simulink library "FVT_lib"  (R2021b)
settings: Solver=VariableStepAuto  StartTime=0.0  StopTime=10.0  RelTol=1e-3
undefined symbols (not defined in the file): C_TASK_5MS_S, CANFDArray, ENUM_FAULTSTATE_FAIL, ENUM_FAULTSTATE_INDETERMINATE, ENUM_FAULTSTATE_PASS, EPSILON, FALSE, KHAL_CounterMAX_enum, KHAL_CounterMAXE2E_enum, LINArray, ONE_INT, TRUE, UNKNOWN, XX2KXX, ZERO_FLOAT, ZERO_INT
libraries: hdlsllib x41, simulink x23, hcu_lib x7, $bdroot x2
(part 2 of 3)

== system FVT_lib/hal/LIN_Scheduler ==
  Chart1 : Stateflow chart  TreatAsAtomicUnit=on
  Constant1 : Constant  Value=C_TASK_5MS_S
  Constant2 : Constant  Value=FirstDelayTime
  Constant3 : Constant  Value=C_TASK_5MS_S
  Constant4 : Constant  Value=CycleTime
  Data Type Conversion : DataTypeConversion  OutDataTypeStr=uint16
  Data Type Conversion1 : DataTypeConversion  OutDataTypeStr=uint16
  Divide : Product  Inputs=*/
  Divide1 : Product  Inputs=*/
  Gain : Gain  Gain=0.001
  Gain1 : Gain  Gain=0.001
  trig_LINReq : Outport
  wires:
  Data Type Conversion/1 -> Chart1/1(CycleCounter)
  Divide/1 -> Data Type Conversion1/1
  Chart1/1(trig_LINReq()) -> trig_LINReq/1
  Constant1/1 -> Divide/2
  Constant3/1 -> Divide1/2
  Divide1/1 -> Data Type Conversion/1
  Data Type Conversion1/1 -> Chart1/2(FirstDelayCounter)
  Constant4/1 -> Gain/1
  Gain/1 -> Divide1/1
  Constant2/1 -> Gain1/1
  Gain1/1 -> Divide/1

== system FVT_lib/hal/MessageRollingCounter ==
  Constant : Constant  Value=task_time_ms  OutDataTypeStr=uint16
  Constant1 : Constant  Value=msg_time_ms  OutDataTypeStr=uint16
  Constant2 : Constant  Value=ONE_INT
  Data Type Conversion : DataTypeConversion  OutDataTypeStr=uint16
  Data Type Conversion1 : DataTypeConversion  OutDataTypeStr=uint16
  Divide : Product  Inputs=*/  OutDataTypeStr=uint16
  Max : MinMax  Function=max  Inputs=2
  Scheduler : Stateflow chart  TreatAsAtomicUnit=on
  Subsystem : Subsystem
  out : Outport
  wires:
  Subsystem/1(RC) -> out/1
  Scheduler/1(trig_counter()) -> Subsystem/Trigger
  Constant1/1 -> Divide/1
  Constant/1 -> Max/1
  Max/1 -> Divide/2
  Constant2/1 -> Data Type Conversion/1
  Data Type Conversion/1 -> Max/2
  Divide/1 -> Data Type Conversion1/1
  Data Type Conversion1/1 -> Scheduler/1(counter_max)

== system FVT_lib/hal/MsgTimeoutJudge_CAN ==
  Rollcnt : Inport
  Constant : Constant  Value=C_TASK_5MS_S
  Constant1 : Constant  Value=1000  OutDataTypeStr=single
  Constant2 : Constant  Value=Gain
  Constant3 : Constant  Value=CycleTime
  Constant4 : Constant  Value=0.001
  DetectChange1 : Subsystem
      mask help: DetectChange
  Equal : RelationalOperator  Operator=>  OutDataTypeStr=boolean  RndMeth=Simplest
  NOT : Logic  Operator=NOT  AllPortsSameDT=off  OutDataTypeStr=boolean
  Product : Product
  Product1 : Product
  Timer1 : Subsystem  mask(Timer){}
      mask help: Timer funcion.
  MsgTimeout_flg : Outport
  wires:
  Rollcnt/1 -> DetectChange1/1(cnt)
  NOT/1 -> Timer1/1(trigger)
  DetectChange1/1(InValid) -> NOT/1, Timer1/2(reset)
  Constant1/1 -> Timer1/4(max_time)
  Constant/1 -> Timer1/3(Ts)
  Constant2/1 -> Product/2
  Product/1 -> Equal/2
  Timer1/1(time) -> Equal/1
  Equal/1 -> MsgTimeout_flg/1
  Constant3/1 -> Product1/1
  Constant4/1 -> Product1/2
  Product1/1 -> Product/1

== system FVT_lib/hal/MsgTimeoutJudge_CAN_AUTOSAR ==
  Cast To Boolean13 : DataTypeConversion  OutDataTypeStr=boolean
  Constant : Constant  Value=TRUE
  Latch13 : hcu_lib/Basic_Blocks/Latch
  Switch13 : Switch  Criteria=u2 ~= 0
  Unit Delay : UnitDelay  SampleTime=-1  HasFrameUpgradeWarning=on
  UnitConverter : DataTypeConversion  OutDataTypeStr=boolean
  Out : Outport
  wires:
  Latch13/1 -> Switch13/2
  Switch13/1 -> UnitConverter/1
  UnitConverter/1 -> Out/1, Unit Delay/1
  Cast To Boolean13/1 -> Latch13/1, Switch13/1
  Unit Delay/1 -> Cast To Boolean13/1
  Constant/1 -> Switch13/3

== system FVT_lib/hal/MsgTimeoutJudge_LIN ==
  Rollcnt : Inport
  Constant2 : Constant  Value=TimeoutCnt
  Data Type Conversion : DataTypeConversion  OutDataTypeStr=uint8
  Data Type Conversion1 : DataTypeConversion  OutDataTypeStr=uint8
  Equal : RelationalOperator  OutDataTypeStr=boolean  RndMeth=Simplest
  MsgTimeout_flg : Outport
  wires:
  Equal/1 -> MsgTimeout_flg/1
  Rollcnt/1 -> Data Type Conversion1/1
  Constant2/1 -> Data Type Conversion/1
  Data Type Conversion/1 -> Equal/2
  Data Type Conversion1/1 -> Equal/1

== system FVT_lib/hal/MsgTxController ==
  TxReq : Inport
  Chart : Stateflow chart  TreatAsAtomicUnit=on
  Constant : Constant  Value=C_TASK_5MS_S
  Constant3 : Constant  Value=CycleTime
  Data Type Conversion : DataTypeConversion  OutDataTypeStr=uint16
  Divide : Product  Inputs=*/
  Gain : Gain  Gain=0.001
  TxTrigger : Outport
  wires:
  Constant/1 -> Divide/2
  TxReq/1 -> Chart/1(TxReq)
  Divide/1 -> Data Type Conversion/1
  Chart/1(TxTrigger()) -> TxTrigger/1
  Gain/1 -> Divide/1
  Constant3/1 -> Gain/1
  Data Type Conversion/1 -> Chart/2(CycleCnt)

== system FVT_lib/hal/MsgTxController_CE ==
  TxReq : Inport
  Signals : Inport  Port=2
  Signals1 : Inport  Port=3
  Chart : Stateflow chart  TreatAsAtomicUnit=on
  Constant : Constant  Value=C_TASK_5MS_S
  Constant3 : Constant  Value=CycleTime
  Data Type Conversion : DataTypeConversion  OutDataTypeStr=uint16
  Divide : Product  Inputs=*/
  Gain : Gain  Gain=0.001
  TxTrigger : Outport
  wires:
  Constant3/1 -> Gain/1
  Gain/1 -> Divide/1
  Chart/1(TxTrigger()) -> TxTrigger/1
  Divide/1 -> Data Type Conversion/1
  Constant/1 -> Divide/2
  [EventReq_flg] -> Chart/2(EventReq)
  TxReq/1 -> Chart/1(TxReq)
  Data Type Conversion/1 -> Chart/3(CycleCnt)

== system FVT_lib/hal/MsgTxController_Event ==
  TxReq : Inport
  Signals : Inport  Port=2
  Signals1 : Inport  Port=3
  Chart : Stateflow chart  TreatAsAtomicUnit=on
  TxTrigger : Outport
  wires:
  TxReq/1 -> Chart/1(TxReq)
  [EventReq_flg] -> Chart/2(EventReq)
  Chart/1(TxTrigger()) -> TxTrigger/1

== system FVT_lib/hal/PutShortSignal ==
  Valfield : Inport
  sfcnSIL_HelpPutSSigWrap : S-Function  FunctionName=sfcnSIL_HelpPutSSigWrap  Parameters=SParameter1, SParameter2, SParameter3  SFunctionDeploymentMode=off  EnableBusSupport=off  mask{SParameter1=SS1-1, SParameter2=SS2, SParameter3=SS3}
      mask prompts: SParameter1 "P1:"; SParameter2 "P2:"; SParameter3 "P3:"
      mask Display: fprintf('Level-2 S-Function SIL_HelpPutSSig');
  wires:
  Valfield/1 -> sfcnSIL_HelpPutSSigWrap/1

== system FVT_lib/hal/RollingCounter ==
  Add2 : Sum
  Constant65 : Constant  Value=CounterMAX
  Constant66 : Constant  Value=ZERO_INT
  Constant67 : Constant  Value=ONE_INT
  Data Type Conversion : DataTypeConversion  OutDataTypeStr=uint8
  Equal34 : RelationalOperator  OutDataTypeStr=boolean  RndMeth=Simplest
  Switch5 : Switch  Criteria=u2 > Threshold
  Unit Delay5 : UnitDelay  SampleTime=-1  HasFrameUpgradeWarning=on
  out : Outport
  wires:
  Switch5/1 -> out/1, Unit Delay5/1
  Equal34/1 -> Switch5/2
  Constant66/1 -> Switch5/1
  Add2/1 -> Switch5/3
  Constant67/1 -> Add2/1
  Unit Delay5/1 -> Equal34/1, Add2/2
  Data Type Conversion/1 -> Equal34/2
  Constant65/1 -> Data Type Conversion/1

== system FVT_lib/hal/RollingCounter_IfAction ==
  CAN_E2E_flg : Inport
  Add2 : Sum
  Constant1 : Constant  Value=KHAL_CounterMAX_enum
  Constant65 : Constant  Value=KHAL_CounterMAXE2E_enum
  Constant66 : Constant  Value=ZERO_INT
  Constant67 : Constant  Value=ONE_INT
  Data Type Conversion : DataTypeConversion  OutDataTypeStr=uint8
  Equal34 : RelationalOperator  OutDataTypeStr=boolean  RndMeth=Simplest
  Switch : Switch  Criteria=u2 ~= 0
  Switch5 : Switch  Criteria=u2 > Threshold
  Unit Delay5 : UnitDelay  SampleTime=-1  HasFrameUpgradeWarning=on
  out : Outport
  wires:
  Unit Delay5/1 -> Add2/2, Equal34/1
  Equal34/1 -> Switch5/2
  Constant66/1 -> Switch5/1
  Data Type Conversion/1 -> Equal34/2
  Constant67/1 -> Add2/1
  Switch/1 -> [CounterMAX]
  CAN_E2E_flg/1 -> Switch/2
  Add2/1 -> Switch5/3
  [CounterMAX] -> Data Type Conversion/1
  Switch5/1 -> Unit Delay5/1, out/1
  Constant1/1 -> Switch/3
  Constant65/1 -> Switch/1

== system FVT_lib/hal/SignalPack ==
  Signal_raw : Inport
  Bitwise AND : simulink/Logic and Bit Operations/Bitwise Operator  logicop=AND  UseBitMask=on  BitMask=BitMask  BitMaskRealWorld=Stored Integer
  Left_shift : ArithShift  BitShiftNumber=LeftShiftCnt  BitShiftDirection=Left
  Right_shift : ArithShift  BitShiftNumber=RightShiftCnt  BitShiftDirection=Right
  out : Outport
  wires:
  Signal_raw/1 -> Right_shift/1
  Right_shift/1 -> Bitwise AND/1
  Bitwise AND/1 -> Left_shift/1
  Left_shift/1 -> out/1

== system FVT_lib/hal/Subsystem ==
  In1 : Inport
  sfcnSIL_HelpPutCSigWrap : S-Function  FunctionName=sfcnSIL_HelpPutCSigWrap  Parameters=SParameter1, SParameter2, SParameter3  SFunctionDeploymentMode=off  EnableBusSupport=off  mask{SParameter1=SS1-1, SParameter2=SS2, SParameter3=SS3}
      mask prompts: SParameter1 "P1:"; SParameter2 "P2:"; SParameter3 "P3:"
      mask Display: fprintf('Level-2 S-Function SIL_HelpPutCSig');
  wires:
  In1/1 -> sfcnSIL_HelpPutCSigWrap/1

== system FVT_lib/hal/convert_in ==
  raw32 : Inport
  Add : Sum
  Data Type Conversion : DataTypeConversion  OutDataTypeStr=single
  Product : Product  RndMeth=Zero
  gain : Constant  Value=single(gain)  OutDataTypeStr=single
  offset : Constant  Value=single(offset)  OutDataTypeStr=single
  value : Outport
  wires:
  raw32/1 -> Data Type Conversion/1
  gain/1 -> Product/2
  Product/1 -> Add/1
  offset/1 -> Add/2
  Add/1 -> value/1
  Data Type Conversion/1 -> Product/1

== system FVT_lib/hal/convert_out ==
  value : Inport
  Add : Sum  Inputs=+-
  Constant : Constant  Value=EPSILON
  Divide : Product  Inputs=*/
  MinMax : MinMax  Function=max  Inputs=2
  gain : Constant  Value=single(gain)  OutDataTypeStr=single
  offset : Constant  Value=single(offset)  OutDataTypeStr=single
  raw32 : Outport
  wires:
  value/1 -> Add/1
  offset/1 -> Add/2
  Add/1 -> Divide/1
  Divide/1 -> raw32/1
  gain/1 -> MinMax/1
  Constant/1 -> MinMax/2
  MinMax/1 -> Divide/2

== system FVT_lib/inp/CAN_Msg_Validity_Process_template ==
  signal_in : Inport
  CAN_Msg_Validity_Process : Subsystem
  debdec : Constant  Value=UNKNOWN
  debinc : Constant  Value=UNKNOWN
  deblim : Constant  Value=UNKNOWN
  inverse : Constant  Value=UNKNOWN
  ovrdflg : Constant  Value=UNKNOWN
  ovrdval : Constant  Value=UNKNOWN
  srvcflg : Constant  Value=UNKNOWN
  srvcval : Constant  Value=UNKNOWN
  signal_out : Outport
  wires:
  signal_in/1 -> CAN_Msg_Validity_Process/1(signal_in)
  CAN_Msg_Validity_Process/1(signal_out) -> signal_out/1
  inverse/1 -> CAN_Msg_Validity_Process/2(inverse_flag)
  deblim/1 -> CAN_Msg_Validity_Process/3(debounce_sat)
  debinc/1 -> CAN_Msg_Validity_Process/4(debounce_inc)
  debdec/1 -> CAN_Msg_Validity_Process/5(debounce_dec)
  ovrdflg/1 -> CAN_Msg_Validity_Process/6(cal_override_flag)
  ovrdval/1 -> CAN_Msg_Validity_Process/7(cal_override_value)
  srvcflg/1 -> CAN_Msg_Validity_Process/8(service_flag)
  srvcval/1 -> CAN_Msg_Validity_Process/9(service_value)

== system FVT_lib/inp/ad_signal_template ==
  signal_raw : Inport
  adc_fault : Inport  Port=2
  vref_fault : Inport  Port=3
  sample_time : Inport  Port=4
  ad_signal_process : Subsystem
  defval : Constant  Value=UNKNOWN
  fftdec : Constant  Value=UNKNOWN
  fftinc : Constant  Value=UNKNOWN
  fftlim : Constant  Value=UNKNOWN
  limlow : Constant  Value=UNKNOWN
  limupr : Constant  Value=UNKNOWN
  ovrdflg : Constant  Value=UNKNOWN
  ovrdval : Constant  Value=UNKNOWN
  srvcflg : Constant  Value=UNKNOWN
  srvcval : Constant  Value=UNKNOWN
  tcfilt : Constant  Value=UNKNOWN
  fault_hi : Outport
  fault_lo : Outport  Port=2
  signal_out : Outport  Port=3
  signal_valid : Outport  Port=4
  wires:
  signal_raw/1 -> ad_signal_process/1(raw_value)
  ad_signal_process/2(signal_range_low_flt) -> fault_lo/1
  ad_signal_process/1(signal_range_high_flt) -> fault_hi/1
  ad_signal_process/4(signal_valid_flg) -> signal_valid/1
  ad_signal_process/3(valid_signal) -> signal_out/1
  limupr/1 -> ad_signal_process/2(raw_upper_limit)
  limlow/1 -> ad_signal_process/3(raw_lower_limit)
  adc_fault/1 -> ad_signal_process/4(adc_fault)
  vref_fault/1 -> ad_signal_process/5(vref_fault)
  sample_time/1 -> ad_signal_process/6(ts)
  tcfilt/1 -> ad_signal_process/7(tc)
  fftlim/1 -> ad_signal_process/8(lim)
  fftinc/1 -> ad_signal_process/9(inc)
  fftdec/1 -> ad_signal_process/10(dec)
  defval/1 -> ad_signal_process/11(def_value)
  ovrdflg/1 -> ad_signal_process/12(cal_ovrdflg)
  ovrdval/1 -> ad_signal_process/13(cal_ovrdval)
  srvcflg/1 -> ad_signal_process/14(service_flag)
  srvcval/1 -> ad_signal_process/15(service_value)

== system FVT_lib/inp/can_signal_template ==
  signal_in : Inport
  signal_valid_in : Inport  Port=2
  msg_valid : Inport  Port=3
  can_signal_process : Subsystem
  defval : Constant  Value=UNKNOWN
  fftdec : Constant  Value=UNKNOWN
  fftinc : Constant  Value=UNKNOWN
  fftlim : Constant  Value=UNKNOWN
  invalid : Constant  Value=UNKNOWN
  ovrdflg : Constant  Value=UNKNOWN
  ovrdval : Constant  Value=UNKNOWN
  setvalid : Constant  Value=UNKNOWN
  srvcflg : Constant  Value=UNKNOWN
  srvcval : Constant  Value=UNKNOWN
  signal_out : Outport
  signal_valid_out : Outport  Port=2
  wires:
  can_signal_process/2(signal_valid_out) -> signal_valid_out/1
  signal_valid_in/1 -> can_signal_process/2(signal_valid_in)
  msg_valid/1 -> can_signal_process/3(msg_valid)
  defval/1 -> can_signal_process/4(default_value)
  fftlim/1 -> can_signal_process/5(fault_filter_lim)
  fftinc/1 -> can_signal_process/6(fault_filter_inc)
  fftdec/1 -> can_signal_process/7(fault_filter_dec)
  invalid/1 -> can_signal_process/8(invalid_override)
  signal_in/1 -> can_signal_process/1(signal_in)
  can_signal_process/1(signal_out) -> signal_out/1
  setvalid/1 -> can_signal_process/9(valid_override)
  ovrdflg/1 -> can_signal_process/10(cal_ovrdflg)
  ovrdval/1 -> can_signal_process/11(cal_ovrdval)
  srvcflg/1 -> can_signal_process/12(service_flag)
  srvcval/1 -> can_signal_process/13(service_value)

== system FVT_lib/inp/di_signal_template ==
  signal_in : Inport
  debdec : Constant  Value=UNKNOWN
  debinc : Constant  Value=UNKNOWN
  deblim : Constant  Value=UNKNOWN
  digital_signal_process : Subsystem  mask(DigitalSignalProcess){}
      mask help: Digital signal process.
  inverse : Constant  Value=UNKNOWN
  ovrdflg : Constant  Value=UNKNOWN
  ovrdval : Constant  Value=UNKNOWN
  srvcflg : Constant  Value=UNKNOWN
  srvcval : Constant  Value=UNKNOWN
  signal_out : Outport
  wires:
  signal_in/1 -> digital_signal_process/1(signal_in)
  digital_signal_process/1(signal_out) -> signal_out/1
  inverse/1 -> digital_signal_process/2(inverse_flag)
  deblim/1 -> digital_signal_process/3(debounce_limit)
  debinc/1 -> digital_signal_process/4(debounce_inc)
  debdec/1 -> digital_signal_process/5(debounce_dec)
  ovrdflg/1 -> digital_signal_process/6(cal_override_flag)
  ovrdval/1 -> digital_signal_process/7(cal_override_value)
  srvcflg/1 -> digital_signal_process/8(service_flag)
  srvcval/1 -> digital_signal_process/9(service_value)

== system FVT_lib/inp/pwm_signal_template ==
  signal_in : Inport
  Constant : Constant  Value=TRUE
  Terminator : Terminator
  override_signal_m1 : Subsystem  TreatAsAtomicUnit=on  RTWFcnName=srvc_ovrd  RTWFileName=HCU_LIB  mask(Override Function){}
      mask help: Override funcion for signal.
      settings: RTWFcnNameOpts=Use subsystem name  RTWFileNameOpts=User specified
  ovrdflg : Constant  Value=UNKNOWN
  ovrdval : Constant  Value=UNKNOWN
  signal_out : Outport
  wires:
  Constant/1 -> override_signal_m1/1(signal_valid_flg_raw)
  override_signal_m1/2(signal_valid_flg) -> Terminator/1
  override_signal_m1/1(signal) -> signal_out/1
  ovrdflg/1 -> override_signal_m1/3(cal_ovrdflg)
  ovrdval/1 -> override_signal_m1/4(cal_ovrdval)
  signal_in/1 -> override_signal_m1/2(signal_raw)

== system FVT_lib/outp/OverrideAndLimit ==
  signal_in : Inport
  Signal_Limit : Subsystem
  Signal_Override : Subsystem
  signal_out : Outport
  wires:
  signal_in/1 -> Signal_Override/1(signal_in)
  Signal_Override/1(signal_out) -> Signal_Limit/1(signal_in)
  Signal_Limit/1(signal_out) -> signal_out/1

== system FVT_lib/hal/CRC8_IfAction_Tx/If Action Subsystem ==
  Byte1 : Inport
  Action Port : ActionPort
  CRC8_Caculation : $bdroot/hal/CRC8_Caculation
  CRC8_Result : Outport
  wires:
  Byte1/1 -> CRC8_Caculation/1
  CRC8_Caculation/1 -> CRC8_Result/1

== system FVT_lib/hal/CRC8_IfAction_Tx/If Action Subsystem1 ==
  CAN_E2E_ID1 : Inport
  CAN_E2E_ID2 : Inport  Port=2
  Byte1 : Inport  Port=3
  Action Port : ActionPort
  CRC8_E2EProfile1 : $bdroot/hal/CRC8_E2EProfile1
  Mux2 : Mux  Inputs=3
  CRC8_E2EResult : Outport
  wires:
  CRC8_E2EProfile1/1 -> CRC8_E2EResult/1
  Byte1/1 -> Mux2/3
  CAN_E2E_ID2/1 -> Mux2/2
  CAN_E2E_ID1/1 -> Mux2/1
  Mux2/1 -> CRC8_E2EProfile1/1

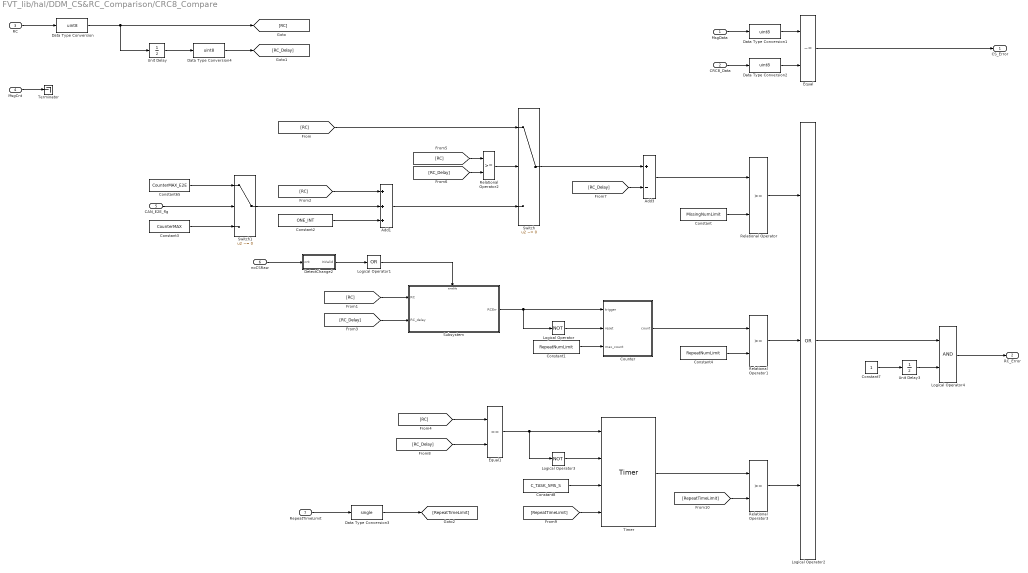
== system FVT_lib/hal/DDM_CS&RC_Comparison/CRC8_Compare ==
  MsgData : Inport
  CRC8_Data : Inport  Port=2
  RC : Inport  Port=3
  MsgCnt : Inport  Port=4
  CAN_E2E_flg : Inport  Port=5
  noCSRaw : Inport  Port=6
  RepeatTimeLimit : Inport  Port=7
  Add1 : Sum  Inputs=+++
  Add3 : Sum  Inputs=+-
  Constant : Constant  Value=MissingNumLimit
  Constant1 : Constant  Value=RepeatNumLimit
  Constant2 : Constant  Value=ONE_INT
  Constant3 : Constant  Value=CounterMAX
  Constant4 : Constant  Value=RepeatNumLimit
  Constant65 : Constant  Value=CounterMAX_E2E
  Constant7 : Constant  OutDataTypeStr=boolean
  Constant8 : Constant  Value=C_TASK_5MS_S
  Counter : Subsystem  mask(Count){}
      mask help: Counter function.
  Data Type Conversion{,1..2,4} (4 alike) : DataTypeConversion  OutDataTypeStr=uint8
  Data Type Conversion3 : DataTypeConversion  OutDataTypeStr=single
  DetectChange2 : Subsystem
      mask help: DetectChange
  Equal : RelationalOperator  Operator=~=  OutDataTypeStr=boolean  RndMeth=Simplest
  Equal1 : RelationalOperator  Operator===  OutDataTypeStr=boolean  RndMeth=Simplest
  Logical Operator : Logic  Operator=NOT  AllPortsSameDT=off  OutDataTypeStr=boolean
  Logical Operator1 : Logic  Operator=OR  Inputs=1  AllPortsSameDT=off  OutDataTypeStr=boolean
  Logical Operator2 : Logic  Operator=OR  Inputs=3  AllPortsSameDT=off  OutDataTypeStr=boolean
  Logical Operator3 : Logic  Operator=NOT  AllPortsSameDT=off  OutDataTypeStr=boolean
  Logical Operator4 : Logic  AllPortsSameDT=off  OutDataTypeStr=boolean
  Relational Operator{,1..3} (4 alike) : RelationalOperator  OutDataTypeStr=boolean  RndMeth=Simplest
  Subsystem : Subsystem
  Switch : Switch  Criteria=u2 ~= 0
  Switch1 : Switch  Criteria=u2 ~= 0
  Terminator : Terminator
  Timer : hcu_lib/Basic_Blocks/Timer
  Unit Delay : UnitDelay  SampleTime=-1  HasFrameUpgradeWarning=on
  Unit Delay3 : UnitDelay  SampleTime=-1  HasFrameUpgradeWarning=on
  CS_Error : Outport
  RC_Error : Outport  Port=2
  wires:
  Equal/1 -> CS_Error/1
  MsgData/1 -> Data Type Conversion1/1
  CRC8_Data/1 -> Data Type Conversion2/1
  Unit Delay/1 -> Data Type Conversion4/1
  Constant/1 -> Relational Operator/2
  Relational Operator/1 -> Logical Operator2/1
  Constant1/1 -> Counter/3(max_count)
  Logical Operator/1 -> Counter/2(reset)
  [RC] -> Add1/1
  Add1/1 -> Switch/3
  RC/1 -> Data Type Conversion/1
  Data Type Conversion/1 -> Unit Delay/1, [RC]
  Constant65/1 -> Switch1/1
  Constant3/1 -> Switch1/3
  Switch1/1 -> Add1/2
  CAN_E2E_flg/1 -> Switch1/2
  Constant2/1 -> Add1/3
  Counter/1(count) -> Relational Operator1/1
  Constant4/1 -> Relational Operator1/2
  Relational Operator1/1 -> Logical Operator2/2
  MsgCnt/1 -> Terminator/1
  Data Type Conversion1/1 -> Equal/1
  Data Type Conversion2/1 -> Equal/2
  Unit Delay3/1 -> Logical Operator4/2
  Constant7/1 -> Unit Delay3/1
  Logical Operator2/1 -> Logical Operator4/1
  Logical Operator4/1 -> RC_Error/1
  Data Type Conversion4/1 -> [RC_Delay]
  [RC] -> Relational Operator2/1
  [RC_Delay] -> Relational Operator2/2
  Relational Operator2/1 -> Switch/2
  [RC] -> Switch/1
  Add3/1 -> Relational Operator/1
  [RC_Delay] -> Add3/2
  Switch/1 -> Add3/1
  Subsystem/1(RCErr) -> Logical Operator/1, Counter/1(trigger)
  [RC] -> Subsystem/1(RC)
  [RC_Delay] -> Subsystem/2(RC_delay)
  noCSRaw/1 -> DetectChange2/1(cnt)
  DetectChange2/1(InValid) -> Logical Operator1/1
  Equal1/1 -> Timer/1, Logical Operator3/1
  [RC_Delay] -> Equal1/2
  [RC] -> Equal1/1
  Timer/1 -> Relational Operator3/1
  Logical Operator3/1 -> Timer/2
  [RepeatTimeLimit] -> Relational Operator3/2
  [RepeatTimeLimit] -> Timer/4
  Constant8/1 -> Timer/3
  Relational Operator3/1 -> Logical Operator2/3
  RepeatTimeLimit/1 -> Data Type Conversion3/1
  Data Type Conversion3/1 -> [RepeatTimeLimit]
  Logical Operator1/1 -> Subsystem/Enable

== system FVT_lib/hal/DDM_CS&RC_Comparison/CRC8_IfAction_Rx ==
  CAN_E2E_flg : Inport
  CAN_E2E_ID1 : Inport  Port=2
  CAN_E2E_ID2 : Inport  Port=3
  Raw : Inport  Port=4
  Data Type Conversion : DataTypeConversion  OutDataTypeStr=uint8
  If : If
  If Action Subsystem : Subsystem  TreatAsAtomicUnit=on
  If Action Subsystem1 : Subsystem  TreatAsAtomicUnit=on
  Merge : Merge
  CRC8 : Outport
  wires:
  If/2 -> If Action Subsystem/Action
  [CAN_E2E_ID1] -> If Action Subsystem1/1(CAN_E2E_ID1)
  [CAN_E2E_ID2] -> If Action Subsystem1/2(CAN_E2E_ID2)
  [Raw] -> If Action Subsystem1/3(Raw)
  If/1 -> If Action Subsystem1/Action
  [Raw] -> If Action Subsystem/1(Raw)
  Data Type Conversion/1 -> If/1
  Merge/1 -> CRC8/1
  If Action Subsystem/1(CRC8_Result) -> Merge/2
  If Action Subsystem1/1(CRC8_E2EResult) -> Merge/1
  [CAN_E2E_flg] -> Data Type Conversion/1
  Raw/1 -> [Raw]
  CAN_E2E_ID2/1 -> [CAN_E2E_ID2]
  CAN_E2E_ID1/1 -> [CAN_E2E_ID1]
  CAN_E2E_flg/1 -> [CAN_E2E_flg]

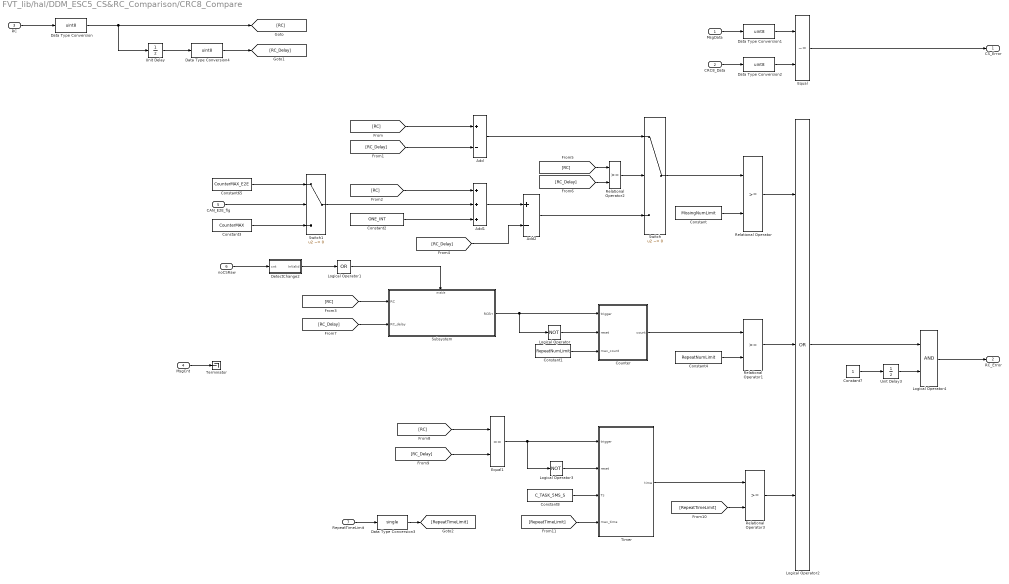
== system FVT_lib/hal/DDM_ESC5_CS&RC_Comparison/CRC8_Compare ==
  MsgData : Inport
  CRC8_Data : Inport  Port=2
  RC : Inport  Port=3
  MsgCnt : Inport  Port=4
  CAN_E2E_flg : Inport  Port=5
  noCSRaw : Inport  Port=6
  RepeatTimeLimit : Inport  Port=7
  Add : Sum  Inputs=+-
  Add1 : Sum  Inputs=+++
  Add2 : Sum  Inputs=+-
  Constant : Constant  Value=MissingNumLimit
  Constant1 : Constant  Value=RepeatNumLimit
  Constant2 : Constant  Value=ONE_INT
  Constant3 : Constant  Value=CounterMAX
  Constant4 : Constant  Value=RepeatNumLimit
  Constant65 : Constant  Value=CounterMAX_E2E
  Constant7 : Constant  OutDataTypeStr=boolean
  Constant8 : Constant  Value=C_TASK_5MS_S
  Counter : Subsystem  mask(Count){}
      mask help: Counter function.
  Data Type Conversion{,1..2,4} (4 alike) : DataTypeConversion  OutDataTypeStr=uint8
  Data Type Conversion3 : DataTypeConversion  OutDataTypeStr=single
  DetectChange2 : Subsystem
      mask help: DetectChange
  Equal : RelationalOperator  Operator=~=  OutDataTypeStr=boolean  RndMeth=Simplest
  Equal1 : RelationalOperator  Operator===  OutDataTypeStr=boolean  RndMeth=Simplest
  Logical Operator : Logic  Operator=NOT  AllPortsSameDT=off  OutDataTypeStr=boolean
  Logical Operator1 : Logic  Operator=OR  Inputs=1  AllPortsSameDT=off  OutDataTypeStr=boolean
  Logical Operator2 : Logic  Operator=OR  Inputs=3  AllPortsSameDT=off  OutDataTypeStr=boolean
  Logical Operator3 : Logic  Operator=NOT  AllPortsSameDT=off  OutDataTypeStr=boolean
  Logical Operator4 : Logic  AllPortsSameDT=off  OutDataTypeStr=boolean
  Relational Operator{,1..3} (4 alike) : RelationalOperator  OutDataTypeStr=boolean  RndMeth=Simplest
  Subsystem : Subsystem
  Switch : Switch  Criteria=u2 ~= 0
  Switch1 : Switch  Criteria=u2 ~= 0
  Terminator : Terminator
  Timer : Subsystem  mask(Timer){}
      mask help: Timer funcion.
  Unit Delay : UnitDelay  SampleTime=-1  HasFrameUpgradeWarning=on
  Unit Delay3 : UnitDelay  SampleTime=-1  HasFrameUpgradeWarning=on
  CS_Error : Outport
  RC_Error : Outport  Port=2
  wires:
  Relational Operator2/1 -> Switch/2
  [RC_Delay] -> Relational Operator2/2
  [RC] -> Relational Operator2/1
  Data Type Conversion4/1 -> [RC_Delay]
  Logical Operator4/1 -> RC_Error/1
  Logical Operator2/1 -> Logical Operator4/1
  Constant7/1 -> Unit Delay3/1
  Unit Delay3/1 -> Logical Operator4/2
  Data Type Conversion2/1 -> Equal/2
  Data Type Conversion1/1 -> Equal/1
  Constant2/1 -> Add1/3
  CAN_E2E_flg/1 -> Switch1/2
  Switch1/1 -> Add1/2
  Constant3/1 -> Switch1/3
  Constant65/1 -> Switch1/1
  Data Type Conversion/1 -> [RC], Unit Delay/1
  RC/1 -> Data Type Conversion/1
  Add2/1 -> Switch/3
  [RC_Delay] -> Add2/2
  Add1/1 -> Add2/1
  [RC] -> Add1/1
  [RC_Delay] -> Add/2
  [RC] -> Add/1
  Add/1 -> Switch/1
  Relational Operator/1 -> Logical Operator2/1
  Constant/1 -> Relational Operator/2
  Switch/1 -> Relational Operator/1
  Unit Delay/1 -> Data Type Conversion4/1
  CRC8_Data/1 -> Data Type Conversion2/1
  MsgData/1 -> Data Type Conversion1/1
  Equal/1 -> CS_Error/1
  Counter/1(count) -> Relational Operator1/1
  Constant1/1 -> Counter/3(max_count)
  Constant4/1 -> Relational Operator1/2
  DetectChange2/1(InValid) -> Logical Operator1/1
  [RC_Delay] -> Subsystem/2(RC_delay)
  Subsystem/1(RCErr) -> Logical Operator/1, Counter/1(trigger)
  Logical Operator3/1 -> Timer/2(reset)
  [RepeatTimeLimit] -> Relational Operator3/2
  [RepeatTimeLimit] -> Timer/4(max_time)
  Equal1/1 -> Timer/1(trigger), Logical Operator3/1
  [RC_Delay] -> Equal1/2
  Timer/1(time) -> Relational Operator3/1
  Constant8/1 -> Timer/3(Ts)
  Logical Operator/1 -> Counter/2(reset)
  [RC] -> Subsystem/1(RC)
  RepeatTimeLimit/1 -> Data Type Conversion3/1
  Relational Operator1/1 -> Logical Operator2/2
  [RC] -> Equal1/1
  noCSRaw/1 -> DetectChange2/1(cnt)
  Relational Operator3/1 -> Logical Operator2/3
  MsgCnt/1 -> Terminator/1
  Data Type Conversion3/1 -> [RepeatTimeLimit]
  Logical Operator1/1 -> Subsystem/Enable

== system FVT_lib/hal/DDM_ESC5_CS&RC_Comparison/CRC8_IfAction_Rx ==
  CAN_E2E_flg : Inport
  CAN_E2E_ID1 : Inport  Port=2
  CAN_E2E_ID2 : Inport  Port=3
  Raw : Inport  Port=4
  Data Type Conversion : DataTypeConversion  OutDataTypeStr=uint8
  If : If
  If Action Subsystem : Subsystem  TreatAsAtomicUnit=on
  If Action Subsystem1 : Subsystem  TreatAsAtomicUnit=on
  Merge : Merge
  CRC8 : Outport
  wires:
  CAN_E2E_flg/1 -> [CAN_E2E_flg]
  CAN_E2E_ID1/1 -> [CAN_E2E_ID1]
  CAN_E2E_ID2/1 -> [CAN_E2E_ID2]
  Raw/1 -> [Raw]
  [CAN_E2E_flg] -> Data Type Conversion/1
  If Action Subsystem1/1(CRC8_E2EResult) -> Merge/1
  If Action Subsystem/1(CRC8_Result) -> Merge/2
  Merge/1 -> CRC8/1
  Data Type Conversion/1 -> If/1
  [Raw] -> If Action Subsystem/1(Raw)
  If/1 -> If Action Subsystem1/Action
  [Raw] -> If Action Subsystem1/3(Raw)
  [CAN_E2E_ID2] -> If Action Subsystem1/2(CAN_E2E_ID2)
  [CAN_E2E_ID1] -> If Action Subsystem1/1(CAN_E2E_ID1)
  If/2 -> If Action Subsystem/Action

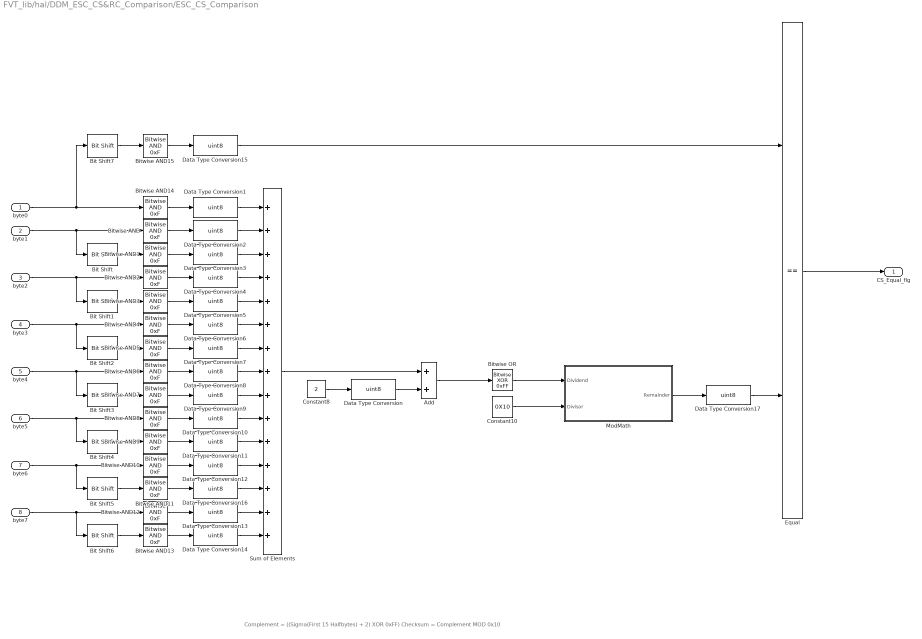
== system FVT_lib/hal/DDM_ESC_CS&RC_Comparison/ESC_CS_Comparison ==
  note: Complement = ((Sigma(First 15 Halfbytes) + 2) XOR 0xFF)
      | Checksum = Complement MOD 0x10
  byte0 : Inport
  byte1 : Inport  Port=2
  byte2 : Inport  Port=3
  byte3 : Inport  Port=4
  byte4 : Inport  Port=5
  byte5 : Inport  Port=6
  byte6 : Inport  Port=7
  byte7 : Inport  Port=8
  Add : Sum
  Bit Shift{,1..7} (8 alike) : hdlsllib/Logic and Bit Operations/Bit Shift  mode=Shift Right Logical  N=4
  Bitwise AND{,1..15} (16 alike) : simulink/Logic and Bit Operations/Bitwise Operator  logicop=AND  UseBitMask=on  BitMask=0xF  BitMaskRealWorld=Stored Integer
  Bitwise OR : simulink/Logic and Bit Operations/Bitwise Operator  logicop=XOR  UseBitMask=on  BitMask=0xFF  BitMaskRealWorld=Stored Integer
  Constant10 : Constant  Value=0X10
  Constant8 : Constant  Value=2  OutDataTypeStr=uint8
  Data Type Conversion{,1..17} (18 alike) : DataTypeConversion  OutDataTypeStr=uint8
  Equal : RelationalOperator  Operator===  OutDataTypeStr=boolean  RndMeth=Simplest
  ModMath : Subsystem  mask(Count){}
      mask help: Counter function.
      mask Display:
      | fprintf('ModMath');
      | port_label('output', 1, 'Remainder');
      | port_label('input', 1, 'Dividend');
      | port_label('input', 2, 'Divisor');
  Sum of Elements : Sum  Inputs=+++++++++++++++
  CS_Equal_flg : Outport
  wires:
  Bitwise AND3/1 -> Data Type Conversion5/1
  Data Type Conversion7/1 -> Sum of Elements/7
  Bitwise AND1/1 -> Data Type Conversion3/1
  Data Type Conversion6/1 -> Sum of Elements/6
  byte3/1 -> Bitwise AND4/1, Bit Shift2/1
  Sum of Elements/1 -> Add/1
  Bitwise AND7/1 -> Data Type Conversion9/1
  Data Type Conversion16/1 -> Sum of Elements/13
  Data Type Conversion1/1 -> Sum of Elements/1
  Data Type Conversion5/1 -> Sum of Elements/5
  Bitwise AND11/1 -> Data Type Conversion16/1
  Bitwise AND5/1 -> Data Type Conversion7/1
  Equal/1 -> CS_Equal_flg/1
  Bitwise AND13/1 -> Data Type Conversion14/1
  Data Type Conversion13/1 -> Sum of Elements/14
  byte7/1 -> Bitwise AND12/1, Bit Shift6/1
  Data Type Conversion15/1 -> Equal/1
  Data Type Conversion12/1 -> Sum of Elements/12
  Bitwise AND14/1 -> Data Type Conversion1/1
  Bit Shift6/1 -> Bitwise AND13/1
  Data Type Conversion11/1 -> Sum of Elements/11
  Bit Shift5/1 -> Bitwise AND11/1
  Data Type Conversion4/1 -> Sum of Elements/4
  Constant10/1 -> ModMath/2(Divisor)
  Constant8/1 -> Data Type Conversion/1
  Data Type Conversion10/1 -> Sum of Elements/10
  Bitwise AND6/1 -> Data Type Conversion8/1
  Data Type Conversion8/1 -> Sum of Elements/8
  Bitwise AND2/1 -> Data Type Conversion4/1
  byte0/1 -> Bitwise AND14/1, Bit Shift7/1
  Bitwise AND15/1 -> Data Type Conversion15/1
  byte6/1 -> Bitwise AND10/1, Bit Shift5/1
  Bit Shift/1 -> Bitwise AND1/1
  Data Type Conversion3/1 -> Sum of Elements/3
  Data Type Conversion14/1 -> Sum of Elements/15
  Data Type Conversion/1 -> Add/2
  byte5/1 -> Bitwise AND8/1, Bit Shift4/1
  Bit Shift7/1 -> Bitwise AND15/1
  Bitwise AND9/1 -> Data Type Conversion11/1
  Bit Shift1/1 -> Bitwise AND3/1
  Bitwise AND/1 -> Data Type Conversion2/1
  Bitwise AND10/1 -> Data Type Conversion12/1
  Bitwise AND12/1 -> Data Type Conversion13/1
  Data Type Conversion9/1 -> Sum of Elements/9
  Bit Shift4/1 -> Bitwise AND9/1
  Data Type Conversion2/1 -> Sum of Elements/2
  Bitwise OR/1 -> ModMath/1(Dividend)
  Bitwise AND8/1 -> Data Type Conversion10/1
  byte4/1 -> Bitwise AND6/1, Bit Shift3/1
  Bit Shift3/1 -> Bitwise AND7/1
  Bit Shift2/1 -> Bitwise AND5/1
  byte1/1 -> Bitwise AND/1, Bit Shift/1
  Add/1 -> Bitwise OR/1
  Bitwise AND4/1 -> Data Type Conversion6/1
  byte2/1 -> Bitwise AND2/1, Bit Shift1/1
  ModMath/1(Remainder) -> Data Type Conversion17/1
  Data Type Conversion17/1 -> Equal/2

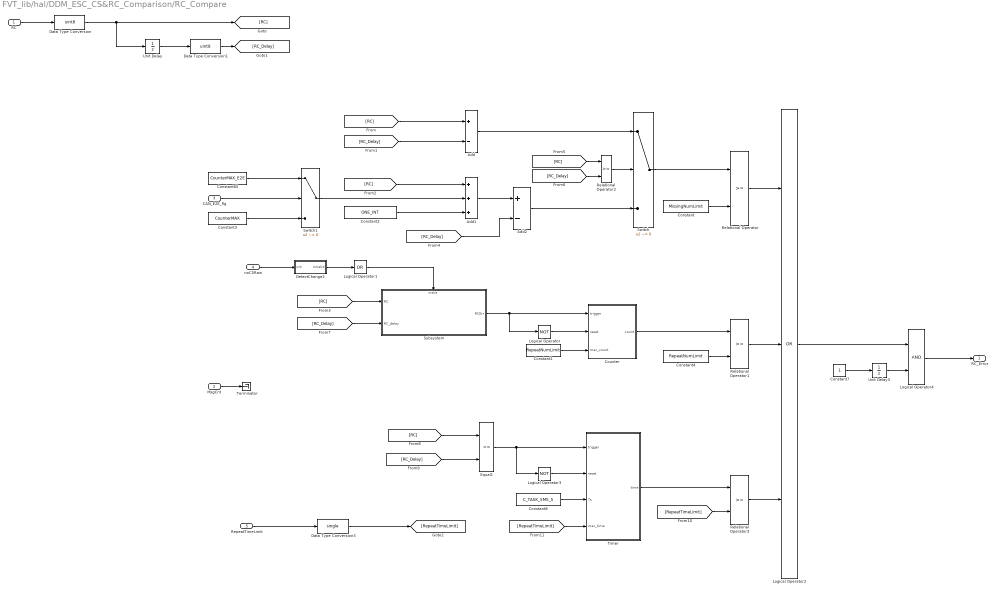
== system FVT_lib/hal/DDM_ESC_CS&RC_Comparison/RC_Compare ==
  RC : Inport
  MsgCnt : Inport  Port=2
  CAN_E2E_flg : Inport  Port=3
  noCSRaw : Inport  Port=4
  RepeatTimeLimit : Inport  Port=5
  Add : Sum  Inputs=+-
  Add1 : Sum  Inputs=+++
  Add2 : Sum  Inputs=+-
  Constant : Constant  Value=MissingNumLimit
  Constant1 : Constant  Value=RepeatNumLimit
  Constant2 : Constant  Value=ONE_INT
  Constant3 : Constant  Value=CounterMAX
  Constant4 : Constant  Value=RepeatNumLimit
  Constant65 : Constant  Value=CounterMAX_E2E
  Constant7 : Constant  OutDataTypeStr=boolean
  Constant8 : Constant  Value=C_TASK_5MS_S
  Counter : Subsystem  mask(Count){}
      mask help: Counter function.
  Data Type Conversion : DataTypeConversion  OutDataTypeStr=uint8
  Data Type Conversion1 : DataTypeConversion  OutDataTypeStr=uint8
  Data Type Conversion3 : DataTypeConversion  OutDataTypeStr=single
  DetectChange2 : Subsystem
      mask help: DetectChange
  Equal1 : RelationalOperator  Operator===  OutDataTypeStr=boolean  RndMeth=Simplest
  Logical Operator : Logic  Operator=NOT  AllPortsSameDT=off  OutDataTypeStr=boolean
  Logical Operator1 : Logic  Operator=OR  Inputs=1  AllPortsSameDT=off  OutDataTypeStr=boolean
  Logical Operator2 : Logic  Operator=OR  Inputs=3  AllPortsSameDT=off  OutDataTypeStr=boolean
  Logical Operator3 : Logic  Operator=NOT  AllPortsSameDT=off  OutDataTypeStr=boolean
  Logical Operator4 : Logic  AllPortsSameDT=off  OutDataTypeStr=boolean
  Relational Operator{,1..3} (4 alike) : RelationalOperator  OutDataTypeStr=boolean  RndMeth=Simplest
  Subsystem : Subsystem
  Switch : Switch  Criteria=u2 ~= 0
  Switch1 : Switch  Criteria=u2 ~= 0
  Terminator : Terminator
  Timer : Subsystem  mask(Timer){}
      mask help: Timer funcion.
  Unit Delay : UnitDelay  SampleTime=-1  HasFrameUpgradeWarning=on
  Unit Delay3 : UnitDelay  SampleTime=-1  HasFrameUpgradeWarning=on
  RC_Error : Outport
  wires:
  Logical Operator4/1 -> RC_Error/1
  Logical Operator2/1 -> Logical Operator4/1
  Constant7/1 -> Unit Delay3/1
  Unit Delay3/1 -> Logical Operator4/2
  Constant2/1 -> Add1/3
  CAN_E2E_flg/1 -> Switch1/2
  Switch1/1 -> Add1/2
  Constant3/1 -> Switch1/3
  Constant65/1 -> Switch1/1
  Data Type Conversion/1 -> [RC], Unit Delay/1
  RC/1 -> Data Type Conversion/1
  Add2/1 -> Switch/3
  [RC_Delay] -> Add2/2
  Add1/1 -> Add2/1
  [RC] -> Add1/1
  [RC_Delay] -> Add/2
  [RC] -> Add/1
  Add/1 -> Switch/1
  Relational Operator/1 -> Logical Operator2/1
  Constant/1 -> Relational Operator/2
  Switch/1 -> Relational Operator/1
  Unit Delay/1 -> Data Type Conversion1/1
  Data Type Conversion1/1 -> [RC_Delay]
  [RC] -> Relational Operator2/1
  [RC_Delay] -> Relational Operator2/2
  Relational Operator2/1 -> Switch/2
  Logical Operator3/1 -> Timer/2(reset)
  Subsystem/1(RCErr) -> Logical Operator/1, Counter/1(trigger)
  noCSRaw/1 -> DetectChange2/1(cnt)
  DetectChange2/1(InValid) -> Logical Operator1/1
  [RC_Delay] -> Subsystem/2(RC_delay)
  Constant4/1 -> Relational Operator1/2
  Counter/1(count) -> Relational Operator1/1
  Logical Operator/1 -> Counter/2(reset)
  Constant1/1 -> Counter/3(max_count)
  Relational Operator1/1 -> Logical Operator2/2
  Relational Operator3/1 -> Logical Operator2/3
  [RC] -> Subsystem/1(RC)
  Constant8/1 -> Timer/3(Ts)
  [RC] -> Equal1/1
  [RC_Delay] -> Equal1/2
  Equal1/1 -> Timer/1(trigger), Logical Operator3/1
  Timer/1(time) -> Relational Operator3/1
  [RepeatTimeLimit] -> Relational Operator3/2
  [RepeatTimeLimit] -> Timer/4(max_time)
  MsgCnt/1 -> Terminator/1
  RepeatTimeLimit/1 -> Data Type Conversion3/1
  Data Type Conversion3/1 -> [RepeatTimeLimit]
  Logical Operator1/1 -> Subsystem/Enable

== system FVT_lib/hal/MessageRollingCounter/Subsystem ==
  Trigger : TriggerPort  TriggerType=function-call  VariantControl=(inherit)  PortDimensions=1
  Add2 : Sum
  Constant65 : Constant  Value=CounterMAX
  Constant66 : Constant  Value=ZERO_INT
  Constant67 : Constant  Value=ONE_INT
  Data Type Conversion : DataTypeConversion  OutDataTypeStr=uint8
  Equal34 : RelationalOperator  OutDataTypeStr=boolean  RndMeth=Simplest
  Switch5 : Switch  Criteria=u2 > Threshold
  Unit Delay5 : UnitDelay  SampleTime=-1  HasFrameUpgradeWarning=on
  RC : Outport
  wires:
  Unit Delay5/1 -> Equal34/1, Add2/2
  Equal34/1 -> Switch5/2
  Constant66/1 -> Switch5/1
  Data Type Conversion/1 -> Equal34/2
  Switch5/1 -> Unit Delay5/1, RC/1
  Constant65/1 -> Data Type Conversion/1
  Add2/1 -> Switch5/3
  Constant67/1 -> Add2/1

== system FVT_lib/hal/MsgTimeoutJudge_CAN/DetectChange1 ==
  cnt : Inport
  Delay : Delay  DelayLength=1  InitialCondition=0
  Relational Operator : RelationalOperator  Operator=~=  OutDataTypeStr=boolean  RndMeth=Simplest
  InValid : Outport
  wires:
  Relational Operator/1 -> InValid/1
  Delay/1 -> Relational Operator/2
  cnt/1 -> Relational Operator/1, Delay/1

== system FVT_lib/hal/MsgTimeoutJudge_CAN/Timer1 ==
  note: /* output signal type is single */
  trigger : Inport
  reset : Inport  Port=2
  Ts : Inport  Port=3
  max_time : Inport  Port=4
  Constant1 : Constant  Value=ZERO_FLOAT  OutDataTypeStr=single
  MinMax : MinMax  Inputs=2
  Subtract2 : Sum
  Switch1 : Switch  Criteria=u2 ~= 0
      settings: AttributesFormatString=<%<Criteria>>
  Switch2 : Switch  Criteria=u2 ~= 0
      settings: AttributesFormatString=<%<Criteria>>
  Unit Delay1 : UnitDelay  SampleTime=-1  HasFrameUpgradeWarning=on
      settings: AttributesFormatString=<initial = %<X0>>
  time : Outport
  wires:
  [last_time] -> Subtract2/1
  max_time/1 -> MinMax/1
  Unit Delay1/1 -> [last_time], Switch1/3
  MinMax/1 -> Unit Delay1/1, time/1
  Switch2/1 -> MinMax/2
  Ts/1 -> Subtract2/2
  Switch1/1 -> Switch2/3
  Constant1/1 -> Switch1/1
  reset/1 -> Switch1/2
  trigger/1 -> Switch2/2
  Subtract2/1 -> Switch2/1

== system FVT_lib/inp/CAN_Msg_Validity_Process_template/CAN_Msg_Validity_Process ==
  signal_in : Inport
  inverse_flag : Inport  Port=2
  debounce_sat : Inport  Port=3
  debounce_inc : Inport  Port=4
  debounce_dec : Inport  Port=5
  cal_override_flag : Inport  Port=6
  cal_override_value : Inport  Port=7
  service_flag : Inport  Port=8
  service_value : Inport  Port=9
  AFL : Subsystem
  Ground : Ground
  Ground1 : Ground
  Ground2 : Ground
  Logical Operator : Logic  Operator=NOT  Inputs=1  AllPortsSameDT=off  OutDataTypeStr=boolean
  SRS_HCU_INP_003 : simulink/Model-Wide Utilities/DocBlock  DocumentType=Text
  Switch1 : Switch  Criteria=u2 ~= 0  Threshold=0.5
  Terminator : Terminator
  Terminator1 : Terminator
  Terminator2 : Terminator
  "override_signal_m2 " : Subsystem  TreatAsAtomicUnit=on  RTWFcnName=srvc_ovrd  RTWFileName=HCU_LIB  mask(Override Function with Service){}
      mask help: Override function with service for signal.
      settings: RTWFcnNameOpts=Use subsystem name  RTWFileNameOpts=User specified
  signal_out : Outport  OutDataTypeStr=boolean
  wires:
  Ground2/1 -> AFL/6(MILAction)
  Ground1/1 -> AFL/5(FaultAction)
  debounce_dec/1 -> AFL/4(dec)
  debounce_inc/1 -> AFL/3(inc)
  debounce_sat/1 -> AFL/2(max)
  AFL/2(afl_fam) -> Terminator2/1
  Logical Operator/1 -> Switch1/1
  Switch1/1 -> AFL/1(fault_enum)
  signal_in/1 -> Logical Operator/1, Switch1/3
  inverse_flag/1 -> Switch1/2
  cal_override_value/1 -> "override_signal_m2 "/6(cal_ovrdval)
  cal_override_flag/1 -> "override_signal_m2 "/5(cal_ovrdflg)
  service_value/1 -> "override_signal_m2 "/4(service_ovrdval)
  service_flag/1 -> "override_signal_m2 "/3(service_ovrdflg)
  Ground/1 -> "override_signal_m2 "/1(signal_valid_flg_raw)
  AFL/1(afl_fault) -> "override_signal_m2 "/2(signal_raw)
  "override_signal_m2 "/2(signal_valid_flg) -> Terminator1/1
  AFL/3(afl_lam) -> Terminator/1
  "override_signal_m2 "/1(signal) -> signal_out/1

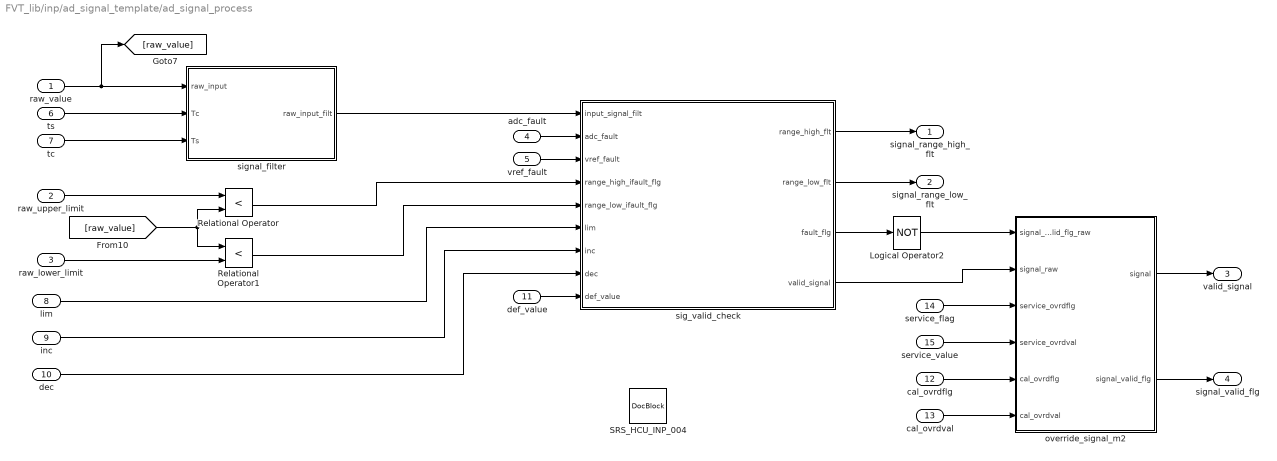
== system FVT_lib/inp/ad_signal_template/ad_signal_process ==
  raw_value : Inport
  raw_upper_limit : Inport  Port=2
  raw_lower_limit : Inport  Port=3
  adc_fault : Inport  Port=4
  vref_fault : Inport  Port=5
  ts : Inport  Port=6
  tc : Inport  Port=7
  lim : Inport  Port=8
  inc : Inport  Port=9
  dec : Inport  Port=10
  def_value : Inport  Port=11
  cal_ovrdflg : Inport  Port=12
  cal_ovrdval : Inport  Port=13
  service_flag : Inport  Port=14
  service_value : Inport  Port=15
  Logical Operator2 : Logic  Operator=NOT  AllPortsSameDT=off  OutDataTypeStr=boolean
  Relational Operator : RelationalOperator  Operator=<  OutDataTypeStr=boolean  RndMeth=Nearest
  Relational Operator1 : RelationalOperator  Operator=<  OutDataTypeStr=boolean  RndMeth=Nearest
  SRS_HCU_INP_004 : simulink/Model-Wide Utilities/DocBlock  DocumentType=Text
  "override_signal_m2 " : Subsystem  TreatAsAtomicUnit=on  RTWFcnName=srvc_ovrd  RTWFileName=HCU_LIB  mask(Override Function with Service){}
      mask help: Override function with service for signal.
      settings: RTWFcnNameOpts=Use subsystem name  RTWFileNameOpts=User specified
  sig_valid_check : Subsystem  RTWFcnName=sig_valid_check
      settings: RTWFcnNameOpts=User specified
  signal_filter : Subsystem
  signal_range_high_flt : Outport
  signal_range_low_flt : Outport  Port=2
  valid_signal : Outport  Port=3
  signal_valid_flg : Outport  Port=4
  wires:
  service_value/1 -> "override_signal_m2 "/4(service_ovrdval)
  vref_fault/1 -> sig_valid_check/3(vref_fault)
  adc_fault/1 -> sig_valid_check/2(adc_fault)
  "override_signal_m2 "/2(signal_valid_flg) -> signal_valid_flg/1
  "override_signal_m2 "/1(signal) -> valid_signal/1
  sig_valid_check/4(valid_signal) -> "override_signal_m2 "/2(signal_raw)
  cal_ovrdval/1 -> "override_signal_m2 "/6(cal_ovrdval)
  cal_ovrdflg/1 -> "override_signal_m2 "/5(cal_ovrdflg)
  service_flag/1 -> "override_signal_m2 "/3(service_ovrdflg)
  sig_valid_check/2(range_low_flt) -> signal_range_low_flt/1
  sig_valid_check/1(range_high_flt) -> signal_range_high_flt/1
  Relational Operator1/1 -> sig_valid_check/5(range_low_ifault_flg)
  signal_filter/1(raw_input_filt) -> sig_valid_check/1(input_signal_filt)
  sig_valid_check/3(fault_flg) -> Logical Operator2/1
  raw_upper_limit/1 -> Relational Operator/1
  raw_lower_limit/1 -> Relational Operator1/2
  lim/1 -> sig_valid_check/6(lim)
  inc/1 -> sig_valid_check/7(inc)
  dec/1 -> sig_valid_check/8(dec)
  def_value/1 -> sig_valid_check/9(def_value)
  [raw_value] -> Relational Operator/2, Relational Operator1/1
  Relational Operator/1 -> sig_valid_check/4(range_high_ifault_flg)
  raw_value/1 -> signal_filter/1(raw_input), [raw_value]
  Logical Operator2/1 -> "override_signal_m2 "/1(signal_valid_flg_raw)
  ts/1 -> signal_filter/2(Tc)
  tc/1 -> signal_filter/3(Ts)

== system FVT_lib/inp/can_signal_template/can_signal_process ==
  signal_in : Inport
  signal_valid_in : Inport  Port=2
  msg_valid : Inport  Port=3
  default_value : Inport  Port=4
  fault_filter_lim : Inport  Port=5
  fault_filter_inc : Inport  Port=6
  fault_filter_dec : Inport  Port=7
  invalid_override : Inport  Port=8
  valid_override : Inport  Port=9
  cal_ovrdflg : Inport  Port=10
  cal_ovrdval : Inport  Port=11
  service_flag : Inport  Port=12
  service_value : Inport  Port=13
  Logical Operator1 : Logic  Operator=NOT  AllPortsSameDT=off  OutDataTypeStr=boolean
  Logical Operator2 : Logic  AllPortsSameDT=off  OutDataTypeStr=boolean
  SRS_HCU_INP_002 : simulink/Model-Wide Utilities/DocBlock  DocumentType=Text
  "override_signal_m2 " : Subsystem  TreatAsAtomicUnit=on  RTWFcnName=srvc_ovrd  RTWFileName=HCU_LIB  mask(Override Function with Service){}
      mask help: Override function with service for signal.
      settings: RTWFcnNameOpts=Use subsystem name  RTWFileNameOpts=User specified
  signal validity checking : Subsystem  TreatAsAtomicUnit=on  RTWFcnName=sig_valid_check  RTWFileName=HCU_LIB  mask(SignalValidCheck){}
      mask help: Signal valid check.
      settings: RTWFcnNameOpts=User specified  RTWFileNameOpts=User specified
  signal_out : Outport
  signal_valid_out : Outport  Port=2
  wires:
  signal validity checking/2(valid_signal) -> "override_signal_m2 "/2(signal_raw)  "valid_flg"
  signal validity checking/1(fault_flg) -> Logical Operator1/1  "fault_flg"
  fault_filter_dec/1 -> signal validity checking/8(dec)
  fault_filter_inc/1 -> signal validity checking/7(inc)
  fault_filter_lim/1 -> signal validity checking/6(sat)
  default_value/1 -> signal validity checking/5(def_value)
  valid_override/1 -> signal validity checking/4(valid_override)
  cal_ovrdval/1 -> "override_signal_m2 "/6(cal_ovrdval)
  cal_ovrdflg/1 -> "override_signal_m2 "/5(cal_ovrdflg)
  service_value/1 -> "override_signal_m2 "/4(service_ovrdval)
  service_flag/1 -> "override_signal_m2 "/3(service_ovrdflg)
  Logical Operator1/1 -> "override_signal_m2 "/1(signal_valid_flg_raw)  "signal_valid_flg_raw"
  invalid_override/1 -> signal validity checking/3(invalid_override)
  Logical Operator2/1 -> signal validity checking/2(new_signal_valid_flg)
  signal_valid_in/1 -> Logical Operator2/1
  signal_in/1 -> signal validity checking/1(new_signal)
  msg_valid/1 -> Logical Operator2/2
  "override_signal_m2 "/1(signal) -> signal_out/1
  "override_signal_m2 "/2(signal_valid_flg) -> signal_valid_out/1

== system FVT_lib/inp/di_signal_template/digital_signal_process ==
  signal_in : Inport
  inverse_flag : Inport  Port=2
  debounce_limit : Inport  Port=3
  debounce_inc : Inport  Port=4
  debounce_dec : Inport  Port=5
  cal_override_flag : Inport  Port=6
  cal_override_value : Inport  Port=7
  service_flag : Inport  Port=8
  service_value : Inport  Port=9
  AFL : Subsystem
  Ground : Ground
  Logical Operator : Logic  Operator=NOT  Inputs=1  AllPortsSameDT=off  OutDataTypeStr=boolean
  Switch1 : Switch  Criteria=u2 ~= 0  Threshold=0.5
  Terminator1 : Terminator
  "override_signal_m2 " : Subsystem  TreatAsAtomicUnit=on  RTWFcnName=srvc_ovrd  RTWFileName=HCU_LIB  mask(Override Function with Service){}
      mask help: Override function with service for signal.
      settings: RTWFcnNameOpts=Use subsystem name  RTWFileNameOpts=User specified
  signal_out : Outport  OutDataTypeStr=boolean
  wires:
  Logical Operator/1 -> Switch1/1
  Switch1/1 -> AFL/1(signal_in)
  signal_in/1 -> Logical Operator/1, Switch1/3
  inverse_flag/1 -> Switch1/2
  cal_override_value/1 -> "override_signal_m2 "/6(cal_ovrdval)
  cal_override_flag/1 -> "override_signal_m2 "/5(cal_ovrdflg)
  service_value/1 -> "override_signal_m2 "/4(service_ovrdval)
  service_flag/1 -> "override_signal_m2 "/3(service_ovrdflg)
  Ground/1 -> "override_signal_m2 "/1(signal_valid_flg_raw)
  AFL/1(afl_fault) -> "override_signal_m2 "/2(signal_raw)
  "override_signal_m2 "/2(signal_valid_flg) -> Terminator1/1
  "override_signal_m2 "/1(signal) -> signal_out/1
  debounce_limit/1 -> AFL/2(debounce_limit)
  debounce_inc/1 -> AFL/3(debounce_inc)
  debounce_dec/1 -> AFL/4(debounce_dec)

== system FVT_lib/inp/pwm_signal_template/override_signal_m1 ==
  note: ONLY ONE ovrdflg (Service_ovrdflg and Cal_ovrdflg) can be valid
      | Set the priority of Service_ovrdflg higher than Cal_ovrdflg
      | In this way, the Cal_ovrd can be automatically disabled in production
  note: When either service_ovrdflg or cal_ovrdflg is true, signal_valid_flg is set as TRUE
  signal_valid_flg_raw : Inport
  signal_raw : Inport  Port=2
  cal_ovrdflg : Inport  Port=3
  cal_ovrdval : Inport  Port=4
  Data Type Duplicate : DataTypeDuplicate  NumInputPorts=3
  Switch1 : Switch  Criteria=u2 ~= 0  Threshold=0.5
  Switch2 : Switch  Criteria=u2 ~= 0  Threshold=0.5
  True : Constant  Value=TRUE  OutDataTypeStr=boolean
  signal : Outport
  signal_valid_flg : Outport  Port=2
  wires:
  Switch1/1 -> Data Type Duplicate/3, signal/1  "signal"
  [cal_ovrdflg] -> Switch2/2
  cal_ovrdflg/1 -> [cal_ovrdflg], Switch1/2  "cal_ovrdflg"
  cal_ovrdval/1 -> Data Type Duplicate/2, Switch1/1  "cal_ovrdval"
  signal_raw/1 -> Data Type Duplicate/1, Switch1/3  "signal_raw"
  True/1 -> Switch2/1
  Switch2/1 -> signal_valid_flg/1  "signal_valid_flg"
  signal_valid_flg_raw/1 -> Switch2/3  "signal_valid_flg_raw"

== system FVT_lib/outp/OverrideAndLimit/Signal_Limit ==
  signal_in : Inport
  Limit : Subsystem  RTWFileName=HCU_LIB  mask(Limit){}
      mask help: Limit funcion.
      settings: RTWFileNameOpts=User specified
  _maxval : Constant  Value=UNKNOWN
  _minval : Constant  Value=UNKNOWN
  signal_out : Outport
  wires:
  _maxval/1 -> Limit/2(upper_limit)
  _minval/1 -> Limit/3(lower_limit)
  signal_in/1 -> Limit/1(input)
  Limit/1(out) -> signal_out/1

== system FVT_lib/outp/OverrideAndLimit/Signal_Override ==
  signal_in : Inport
  Constant5 : Constant  Value=TRUE
  Terminator : Terminator
  _ovrdflg : Constant  Value=UNKNOWN
  _ovrdval : Constant  Value=UNKNOWN
  "override_signal_m2 " : Subsystem  TreatAsAtomicUnit=on  RTWFcnName=srvc_ovrd  RTWFileName=HCU_LIB  mask(Override Function with Service){}
      mask help: Override function with service for signal.
      settings: RTWFcnNameOpts=Use subsystem name  RTWFileNameOpts=User specified
  signal_out : Outport
  wires:
  _ovrdflg/1 -> "override_signal_m2 "/3(cal_ovrdflg)
  _ovrdval/1 -> "override_signal_m2 "/4(cal_ovrdval)
  Constant5/1 -> "override_signal_m2 "/1(signal_valid_flg_raw)
  "override_signal_m2 "/2(signal_valid_flg) -> Terminator/1
  signal_in/1 -> "override_signal_m2 "/2(signal_raw)
  "override_signal_m2 "/1(signal) -> signal_out/1

== system FVT_lib/hal/DDM_CS&RC_Comparison/CRC8_Compare/Counter ==
  note: /* Max Value of counter is 65535 */
  trigger : Inport
  reset : Inport  Port=2
  max_count : Inport  Port=3
  Constant1 : Constant  Value=ZERO_INT  OutDataTypeStr=uint16
  Constant2 : Constant  Value=uint16(1)  OutDataTypeStr=uint16
  Data Type Conversion : DataTypeConversion  OutDataTypeStr=uint16
  MinMax : MinMax  Inputs=2
  Saturation : Saturate  UpperLimit=65535  LowerLimit=0
      settings: AttributesFormatString=<upper = %<UpperLimit>>\n<lower = %<LowerLimit>>
  Subtract2 : Sum
  Switch1 : Switch  Criteria=u2 ~= 0
      settings: AttributesFormatString=<%<Criteria>>
  Switch2 : Switch  Criteria=u2 ~= 0
      settings: AttributesFormatString=<%<Criteria>>
  Unit Delay1 : UnitDelay  SampleTime=-1  HasFrameUpgradeWarning=on
      settings: AttributesFormatString=<initial = %<X0>>
  count : Outport
  wires:
  Saturation/1 -> MinMax/1
  [last_count] -> Subtract2/1
  max_count/1 -> Saturation/1
  Unit Delay1/1 -> Switch2/3, [last_count]
  MinMax/1 -> Data Type Conversion/1
  Constant2/1 -> Subtract2/2
  Constant1/1 -> Switch1/1
  reset/1 -> Switch1/2
  Switch1/1 -> MinMax/2
  Switch2/1 -> Switch1/3
  trigger/1 -> Switch2/2
  Subtract2/1 -> Switch2/1
  Data Type Conversion/1 -> count/1, Unit Delay1/1

== system FVT_lib/hal/DDM_CS&RC_Comparison/CRC8_Compare/DetectChange2 ==
  cnt : Inport
  Constant : Constant  OutDataTypeStr=boolean
  Data Type Conversion3 : DataTypeConversion  OutDataTypeStr=uint8
  Delay : Delay  DelayLength=1  InitialCondition=0
  Delay1 : Delay  DelayLength=1  InitialCondition=0
  Logical Operator : Logic  AllPortsSameDT=off  OutDataTypeStr=boolean
  Relational Operator : RelationalOperator  Operator=~=  OutDataTypeStr=boolean  RndMeth=Simplest
  InValid : Outport
  wires:
  Data Type Conversion3/1 -> Relational Operator/2
  Delay/1 -> Data Type Conversion3/1
  cnt/1 -> Relational Operator/1, Delay/1
  Constant/1 -> Delay1/1
  Delay1/1 -> Logical Operator/2
  Relational Operator/1 -> Logical Operator/1
  Logical Operator/1 -> InValid/1

== system FVT_lib/hal/DDM_CS&RC_Comparison/CRC8_Compare/Subsystem ==
  RC : Inport
  RC_delay : Inport  Port=2
  Enable : EnablePort
  Equal1 : RelationalOperator  Operator===  OutDataTypeStr=boolean  RndMeth=Simplest
  RCErr : Outport
  wires:
  RC/1 -> Equal1/1
  Equal1/1 -> RCErr/1
  RC_delay/1 -> Equal1/2
